simulink library "lca"  (R2013b)
settings: Solver=ode1  StartTime=0.0  StopTime=Inf  FixedStep=0.001  RelTol=1e-3
PostLoadFcn:
  | , if any(exist('dsrtsu_mdlpostloadfcn', 'file') == [2, 3, 6]), try dsrtsu_mdlpostloadfcn('Execute', bdroot); catch fprintf('Error in PostLoadFcn (dsrtsu_mdlpostloadfcn) for model "%s":\n %s\n', bdroot, lasterr); end, end,
undefined symbols (not defined in the file or in its folder): ALCA_VehSpd_X_kph, C_TASK_5MS_S, ENUM_LCASTATE_ADASFAILURE, ENUM_LCASTATE_DISABLED, ENUM_LCASTATE_EPSRECOVERYPENDING, ENUM_LCASTATE_LEFTASSISTING, ENUM_LCASTATE_OFF, ENUM_LCASTATE_OPERATIONAL, ENUM_LCASTATE_RIGHTASSISTING, ENUM_LCASTATE_STANDBY, FALSE, MLCA_ChangeRate_Y_rat, TRUE
libraries: simulink x2, hcu_lib x1
settings Model: DSRTSU_INTERNAL_RTI_VER=450  DSRTSU_INTERNAL_RTI_TYPE=rti1401  RTICANMMDATA=struct('GeneralSetupData',struct('modelroot','C:\ADAS\trunk\ADAS_Softwares\HTDragon\software\sw_development\arch\app\lca','generalsettings',struct('filesettings',struct('destfolder',struct('Name','RTICANMM_FILES','Check',1),'buildfolder',struct('Name','.','Check',1),'AbsDestfolder',struct('Name','C:\ADAS\trunk\ADAS_Softwares\HTDragon\software\sw_development\arch\app\lca\RTICANMM_FILES'),'AbsBuildfolder',struct('Name','C:\ADAS\trunk\ADAS_Softwares\HTDragon\software\sw_development\arch\app\lca'))),'options',struct('addpaths',1,'rmpaths',1,'addtrcexclusion',logical(1),'cannavigator',struct('checkmonitoring',0),'show_usrtrc',0,'use_usrtrc',0),'advanced',struct('options',[1 1 1 1 1 1 1 1 1 1 1 1 1 1 1 1 1 1 1 1 1 1 1 1 1 1 1 1 1 1 1 1 1 1 1 1 1 1 1 1 1 1 1 1 1 1 1 1 1 1 1 1 1 1 1 1 1 1 1 1 1 1 1 1 1 1 1 1 1 1 1 1 1 1 1 1 1 1 1 1 1 1 1 1 1 1 1 1 1 1 1 1 1 1 1 1 1 1 1 1]),'MPSetup',{{}},'modelname','lca','block','lca'))  DSRTSU_INTERNAL_RTIFPGA=40  Creator=13192  LastModifiedBy=13192

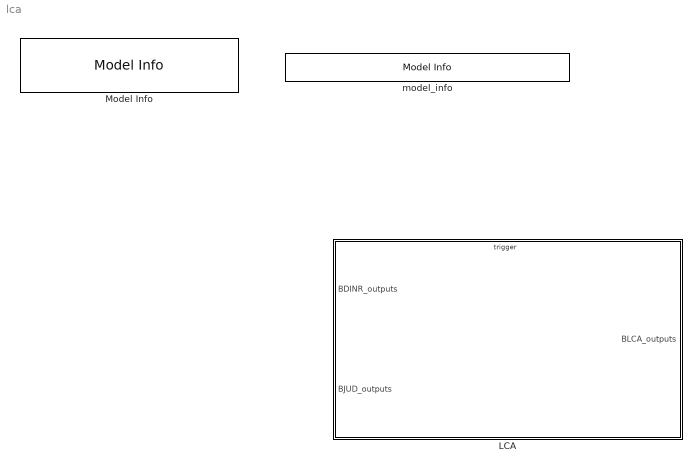
== system lca ==
  LCA : Subsystem
  Model Info : simulink/Model-Wide Utilities/Model Info  InitialBlockCM=None  BlockCM=none  Frame=on  DisplayStringWithTags=|  HorizontalTextAlignment=Left  LeftAlignmentValue=0.02  SourceBlockDiagram=lca  TagMaxNumber=20
      | Model Version        : %<ModelVersion>
      | Creator                   : %<Creator>
      | Last Modified by    : %<LastModifiedBy>
  model_info : simulink/Model-Wide Utilities/Model Info  InitialBlockCM=None  BlockCM=none  Frame=on  DisplayStringWithTags=$Id: hcu_lib.mdl 1464 2016-08-01 05:27:43Z chimotsai $  HorizontalTextAlignment=Center  LeftAlignmentValue=0.5  SourceBlockDiagram=lca  TagMaxNumber=20

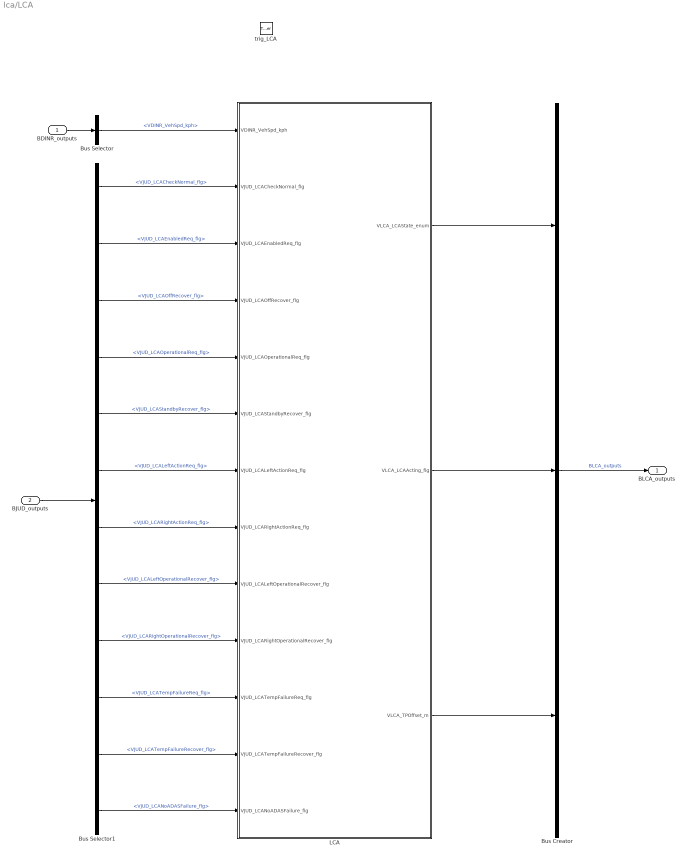
== system lca/LCA ==
  BDINR_outputs : Inport  OutDataTypeStr=Bus: BDINR_outputs
  BJUD_outputs : Inport  Port=2  OutDataTypeStr=Bus: BJUD_outputs
  trig_LCA : TriggerPort  TriggerType=function-call
      settings: AttributesFormatString=State = %<StatesWhenEnabling>
  Bus Creator : BusCreator  Inputs=3  OutDataTypeStr=Bus: BLCA_outputs
  Bus Selector : BusSelector  OutputSignals=VDINR_VehSpd_kph
  Bus Selector1 : BusSelector  OutputSignals=VJUD_LCACheckNormal_flg,VJUD_LCAEnabledReq_flg,VJUD_LCAOffRecover_flg,VJUD_LCAOperationalReq_flg,VJUD_LCAStandbyRecover_flg,VJUD_LCALeftActionReq_flg,VJUD_LCARightActionReq_flg,VJUD_LCALeftOperationalRecover_flg,VJUD_LCARightOperationalRecover_flg,VJUD_LCATempFailureReq_flg,VJUD_LCATempFailureRecover_flg,VJUD_LCANoADASFailure_flg
  LCA : Subsystem
  BLCA_outputs : Outport  OutDataTypeStr=Bus: BLCA_outputs
  wires:
  Bus Selector1/11 -> LCA/12(VJUD_LCATempFailureRecover_flg)  "<VJUD_LCATempFailureRecover_flg>"
  Bus Selector1/12 -> LCA/13(VJUD_LCANoADASFailure_flg)  "<VJUD_LCANoADASFailure_flg>"
  Bus Selector1/10 -> LCA/11(VJUD_LCATempFailureReq_flg)  "<VJUD_LCATempFailureReq_flg>"
  Bus Selector1/9 -> LCA/10(VJUD_LCARightOperationalRecover_flg)  "<VJUD_LCARightOperationalRecover_flg>"
  Bus Selector1/8 -> LCA/9(VJUD_LCALeftOperationalRecover_flg)  "<VJUD_LCALeftOperationalRecover_flg>"
  Bus Selector1/7 -> LCA/8(VJUD_LCARightActionReq_flg)  "<VJUD_LCARightActionReq_flg>"
  Bus Selector1/6 -> LCA/7(VJUD_LCALeftActionReq_flg)  "<VJUD_LCALeftActionReq_flg>"
  Bus Selector1/5 -> LCA/6(VJUD_LCAStandbyRecover_flg)  "<VJUD_LCAStandbyRecover_flg>"
  Bus Selector1/4 -> LCA/5(VJUD_LCAOperationalReq_flg)  "<VJUD_LCAOperationalReq_flg>"
  Bus Selector1/3 -> LCA/4(VJUD_LCAOffRecover_flg)  "<VJUD_LCAOffRecover_flg>"
  Bus Selector1/2 -> LCA/3(VJUD_LCAEnabledReq_flg)  "<VJUD_LCAEnabledReq_flg>"
  Bus Selector1/1 -> LCA/2(VJUD_LCACheckNormal_flg)  "<VJUD_LCACheckNormal_flg>"
  Bus Selector/1 -> LCA/1(VDINR_VehSpd_kph)  "<VDINR_VehSpd_kph>"
  LCA/1(VLCA_LCAState_enum) -> Bus Creator/1
  LCA/3(VLCA_TPOffset_m) -> Bus Creator/3
  LCA/2(VLCA_LCAActing_flg) -> Bus Creator/2
  BJUD_outputs/1 -> Bus Selector1/1
  BDINR_outputs/1 -> Bus Selector/1
  Bus Creator/1 -> BLCA_outputs/1  "BLCA_outputs"

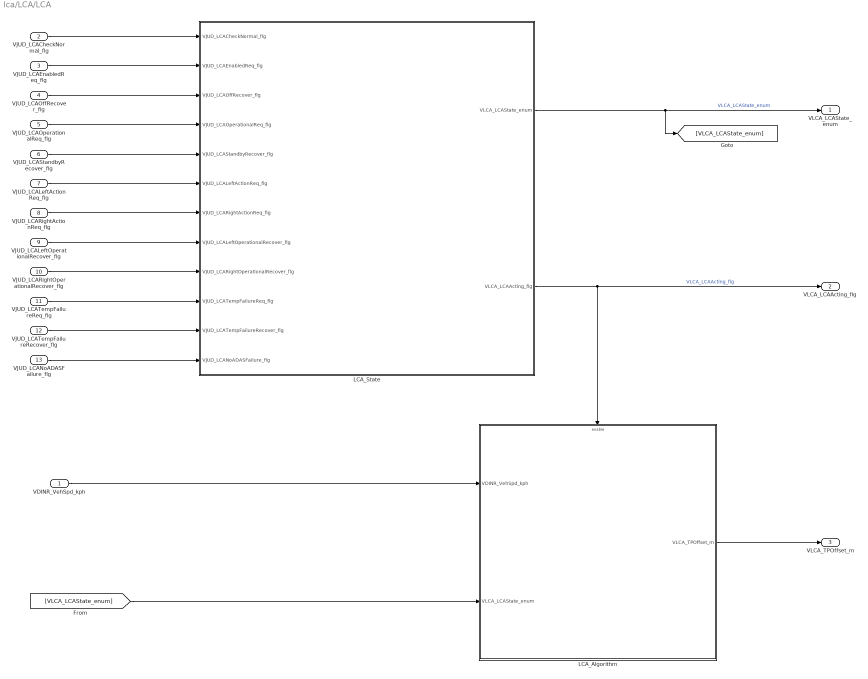
== system lca/LCA/LCA ==
  VDINR_VehSpd_kph : Inport
  VJUD_LCACheckNormal_flg : Inport  Port=2
  VJUD_LCAEnabledReq_flg : Inport  Port=3
  VJUD_LCAOffRecover_flg : Inport  Port=4
  VJUD_LCAOperationalReq_flg : Inport  Port=5
  VJUD_LCAStandbyRecover_flg : Inport  Port=6
  VJUD_LCALeftActionReq_flg : Inport  Port=7
  VJUD_LCARightActionReq_flg : Inport  Port=8
  VJUD_LCALeftOperationalRecover_flg : Inport  Port=9
  VJUD_LCARightOperationalRecover_flg : Inport  Port=10
  VJUD_LCATempFailureReq_flg : Inport  Port=11
  VJUD_LCATempFailureRecover_flg : Inport  Port=12
  VJUD_LCANoADASFailure_flg : Inport  Port=13
  LCA_Algorithm : Subsystem
  LCA_State : Stateflow chart  TreatAsAtomicUnit=on
  VLCA_LCAState_enum : Outport  OutputWhenDisabled=reset  InitialOutput=[0]
  VLCA_LCAActing_flg : Outport  Port=2  OutputWhenDisabled=reset  InitialOutput=[0]
  VLCA_TPOffset_m : Outport  Port=3  OutputWhenDisabled=reset  InitialOutput=[0]
  wires:
  VJUD_LCATempFailureReq_flg/1 -> LCA_State/10(VJUD_LCATempFailureReq_flg)
  [VLCA_LCAState_enum] -> LCA_Algorithm/2(VLCA_LCAState_enum)
  VDINR_VehSpd_kph/1 -> LCA_Algorithm/1(VDINR_VehSpd_kph)
  VJUD_LCARightOperationalRecover_flg/1 -> LCA_State/9(VJUD_LCARightOperationalRecover_flg)
  VJUD_LCARightActionReq_flg/1 -> LCA_State/7(VJUD_LCARightActionReq_flg)
  LCA_Algorithm/1(VLCA_TPOffset_m) -> VLCA_TPOffset_m/1
  LCA_State/2(VLCA_LCAActing_flg) -> LCA_Algorithm/Enable, VLCA_LCAActing_flg/1  "VLCA_LCAActing_flg"
  LCA_State/1(VLCA_LCAState_enum) -> VLCA_LCAState_enum/1, [VLCA_LCAState_enum]  "VLCA_LCAState_enum"
  VJUD_LCANoADASFailure_flg/1 -> LCA_State/12(VJUD_LCANoADASFailure_flg)
  VJUD_LCATempFailureRecover_flg/1 -> LCA_State/11(VJUD_LCATempFailureRecover_flg)
  VJUD_LCALeftOperationalRecover_flg/1 -> LCA_State/8(VJUD_LCALeftOperationalRecover_flg)
  VJUD_LCALeftActionReq_flg/1 -> LCA_State/6(VJUD_LCALeftActionReq_flg)
  VJUD_LCAStandbyRecover_flg/1 -> LCA_State/5(VJUD_LCAStandbyRecover_flg)
  VJUD_LCAOperationalReq_flg/1 -> LCA_State/4(VJUD_LCAOperationalReq_flg)
  VJUD_LCAOffRecover_flg/1 -> LCA_State/3(VJUD_LCAOffRecover_flg)
  VJUD_LCAEnabledReq_flg/1 -> LCA_State/2(VJUD_LCAEnabledReq_flg)
  VJUD_LCACheckNormal_flg/1 -> LCA_State/1(VJUD_LCACheckNormal_flg)

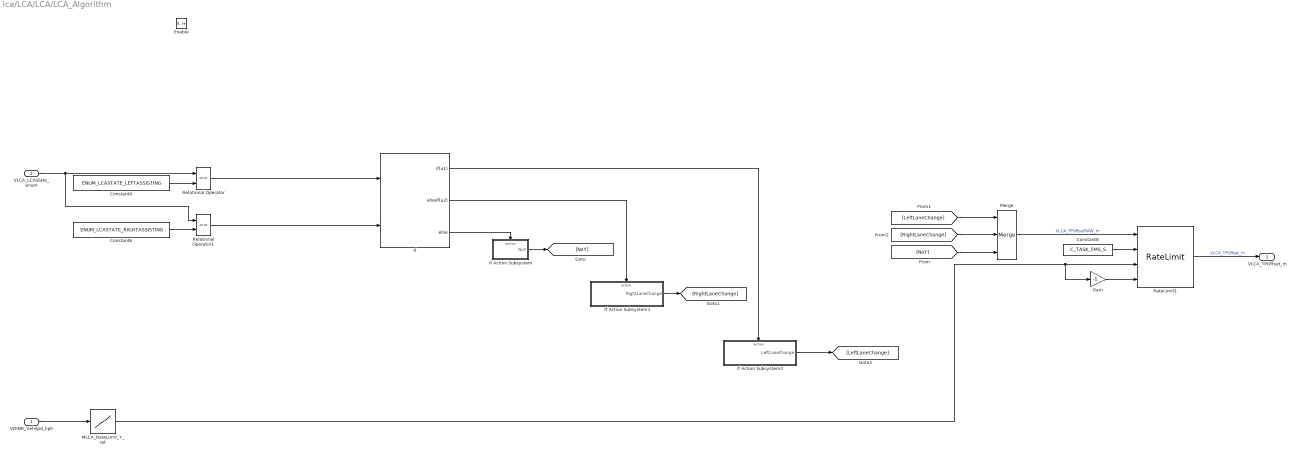
== system lca/LCA/LCA/LCA_Algorithm ==
  VDINR_VehSpd_kph : Inport
  VLCA_LCAState_enum : Inport  Port=2
  Enable : EnablePort  StatesWhenEnabling=reset
  Constant4 : Constant  Value=ENUM_LCASTATE_LEFTASSISTING
  Constant6 : Constant  Value=ENUM_LCASTATE_RIGHTASSISTING
  Constant8 : Constant  Value=C_TASK_5MS_S  OutDataTypeStr=single
  Gain : Gain  Gain=-1
  If : If  NumInputs=2  IfExpression=u1  ElseIfExpressions=u2
  If Action Subsystem : Subsystem  TreatAsAtomicUnit=on
  If Action Subsystem1 : Subsystem  TreatAsAtomicUnit=on
  If Action Subsystem2 : Subsystem  TreatAsAtomicUnit=on
  MLCA_RateLimit_Y_rat : Lookup  InputValues=ALCA_VehSpd_X_kph  Table=MLCA_ChangeRate_Y_rat  LookUpMeth=Interpolation-Use End Values
      settings: AttributesFormatString=%<InputValues>\n%<Table>
  Merge : Merge  Inputs=3
  RateLimit1 : hcu_lib/RateLimit  SystemSampleTime=-1
  Relational Operator : RelationalOperator  Operator===  OutDataTypeStr=boolean
  Relational Operator1 : RelationalOperator  Operator===  OutDataTypeStr=boolean
  VLCA_TPOffset_m : Outport  OutputWhenDisabled=reset  InitialOutput=[0]
  wires:
  RateLimit1/1 -> VLCA_TPOffset_m/1  "VLCA_TPOffset_m"
  Gain/1 -> RateLimit1/4
  Constant8/1 -> RateLimit1/2
  MLCA_RateLimit_Y_rat/1 -> Gain/1, RateLimit1/3
  [RightLaneChange] -> Merge/2
  [LeftLaneChange] -> Merge/1
  [NoY] -> Merge/3
  Merge/1 -> RateLimit1/1  "VLCA_TPOffsetRAW_m"
  If Action Subsystem2/1(LeftLaneChange) -> [LeftLaneChange]
  If Action Subsystem1/1(RightLaneChange) -> [RightLaneChange]
  If Action Subsystem/1(NoY) -> [NoY]
  VDINR_VehSpd_kph/1 -> MLCA_RateLimit_Y_rat/1
  If/3 -> If Action Subsystem/Action
  If/2 -> If Action Subsystem1/Action
  If/1 -> If Action Subsystem2/Action
  Relational Operator1/1 -> If/2
  Constant6/1 -> Relational Operator1/2
  Relational Operator/1 -> If/1
  Constant4/1 -> Relational Operator/2
  VLCA_LCAState_enum/1 -> Relational Operator/1, Relational Operator1/1

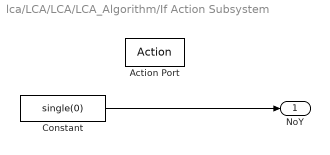
== system lca/LCA/LCA/LCA_Algorithm/If Action Subsystem ==
  Action Port : ActionPort  InitializeStates=reset  ActionType=else
  Constant : Constant  Value=single(0)
  NoY : Outport  InitialOutput=[0]
  wires:
  Constant/1 -> NoY/1

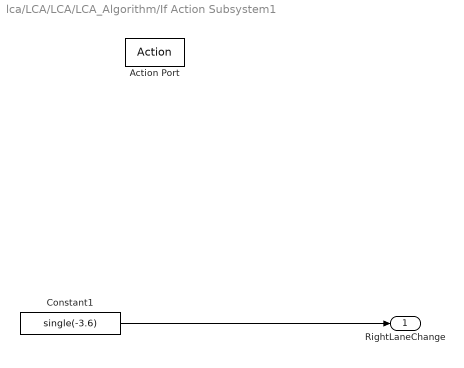
== system lca/LCA/LCA/LCA_Algorithm/If Action Subsystem1 ==
  Action Port : ActionPort  InitializeStates=reset  ActionType=elseif
  Constant1 : Constant  Value=single(-3.6)  OutDataTypeStr=single
  RightLaneChange : Outport  InitialOutput=[0]
  wires:
  Constant1/1 -> RightLaneChange/1

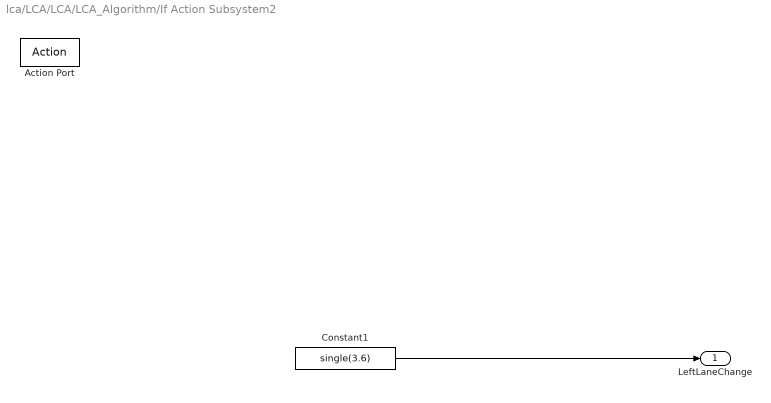
== system lca/LCA/LCA/LCA_Algorithm/If Action Subsystem2 ==
  Action Port : ActionPort  InitializeStates=reset  ActionType=then
  Constant1 : Constant  Value=single(3.6)  OutDataTypeStr=single
  LeftLaneChange : Outport  InitialOutput=[0]
  wires:
  Constant1/1 -> LeftLaneChange/1

== stateflow chart lca/LCA/LCA/LCA_State ==
  state NORMAL
    state ON
      state ENABLED
        state ACTIVE
          state OPERATIONAL
            en:
            VLCA_LCAState_enum=ENUM_LCASTATE_OPERATIONAL;
            VLCA_LCAActing_flg = FALSE;
          state LEFT_ASSIST
            en:
            VLCA_LCAState_enum=ENUM_LCASTATE_LEFTASSISTING;
            VLCA_LCAActing_flg = TRUE;
          state RIGHT_ASSIST
            en:
            VLCA_LCAState_enum=ENUM_LCASTATE_RIGHTASSISTING;
            VLCA_LCAActing_flg = TRUE;
          (default) -> OPERATIONAL
          OPERATIONAL -> LEFT_ASSIST [order 1] : [VJUD_LCALeftActionReq_flg]
          LEFT_ASSIST -> OPERATIONAL : [VJUD_LCALeftOperationalRecover_flg]
          OPERATIONAL -> RIGHT_ASSIST [order 2] : [VJUD_LCARightActionReq_flg]
          RIGHT_ASSIST -> OPERATIONAL : [VJUD_LCARightOperationalRecover_flg]
        state STANDBY
          en:
          VLCA_LCAState_enum=ENUM_LCASTATE_STANDBY;
          VLCA_LCAActing_flg = FALSE;
        (default) -> STANDBY
        STANDBY -> ACTIVE : [VJUD_LCAOperationalReq_flg]
        ACTIVE -> STANDBY : [VJUD_LCAStandbyRecover_flg]
      state OFF
        en:
        VLCA_LCAState_enum=ENUM_LCASTATE_OFF;
        VLCA_LCAActing_flg = FALSE;
      (default) -> OFF
      OFF -> ENABLED : [VJUD_LCAEnabledReq_flg]
      ENABLED -> OFF : [VJUD_LCAOffRecover_flg]
    state DISABLED
      en:
      VLCA_LCAState_enum=ENUM_LCASTATE_DISABLED;
      VLCA_LCAActing_flg = FALSE;
    (default) -> DISABLED
    DISABLED -> ON : [VJUD_LCACheckNormal_flg]
    ON -> DISABLED : [!VJUD_LCACheckNormal_flg]
  state FAILURE_TEMPORARY
    state ADAS_FAILURE
      en:
      VLCA_LCAState_enum=ENUM_LCASTATE_ADASFAILURE;
      VLCA_LCAActing_flg = FALSE;
    state EPS_FAILURE
      en:
      VLCA_LCAState_enum=ENUM_LCASTATE_EPSRECOVERYPENDING;
      VLCA_LCAActing_flg = FALSE;
    (default) -> ADAS_FAILURE
    ADAS_FAILURE -> EPS_FAILURE : [VJUD_LCANoADASFailure_flg]
    EPS_FAILURE -> ADAS_FAILURE : [!VJUD_LCANoADASFailure_flg]
  (default) -> NORMAL
  NORMAL -> FAILURE_TEMPORARY : [VJUD_LCATempFailureReq_flg]
  FAILURE_TEMPORARY -> NORMAL : [VJUD_LCATempFailureRecover_flg]
  data: TRUE parameter; FALSE parameter; ENUM_LCASTATE_DISABLED parameter; ENUM_LCASTATE_OFF parameter; ENUM_LCASTATE_STANDBY parameter; ENUM_LCASTATE_OPERATIONAL parameter; ENUM_LCASTATE_RIGHTASSISTING parameter; ENUM_LCASTATE_ADASFAILURE parameter; ENUM_LCASTATE_EPSRECOVERYPENDING parameter; VLCA_LCAState_enum output double; VLCA_LCAActing_flg output double; VJUD_LCACheckNormal_flg input; VJUD_LCAEnabledReq_flg input; VJUD_LCAOffRecover_flg input; VJUD_LCAOperationalReq_flg input; VJUD_LCAStandbyRecover_flg input; VJUD_LCALeftActionReq_flg input; VJUD_LCARightActionReq_flg input; VJUD_LCALeftOperationalRecover_flg input; VJUD_LCARightOperationalRecover_flg input; VJUD_LCATempFailureReq_flg input; VJUD_LCATempFailureRecover_flg input; VJUD_LCANoADASFailure_flg input; ENUM_LCASTATE_LEFTASSISTING parameter
